simulink model "antywindup"  (R2019a)
settings: Solver=VariableStepAuto  StartTime=0.0  StopTime=50  RelTol=1e-3
values from neighbouring files (symbols this model uses):
  Kc = 10    [skrypt.m]
  Ki = 0.2    [skrypt.m]
  Kp = 2    [skrypt.m]
  u_sat = 10    [skrypt.m]
  y_ref = 10    [skrypt.m]
settings Model: Creator=szymo  LastModifiedBy=szymo

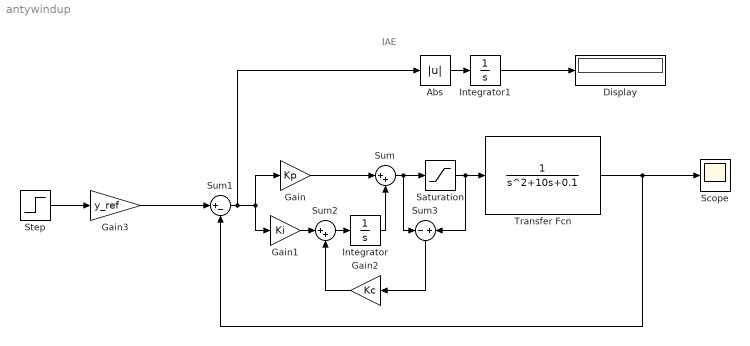
== system antywindup ==
  note: IAE
  Abs : Abs
  Display : Display
  Gain : Gain  Gain=Kp
  Gain1 : Gain  Gain=Ki
  Gain2 : Gain  Gain=Kc
  Gain3 : Gain  Gain=y_ref
  Integrator : Integrator
  Integrator1 : Integrator
  Saturation : Saturate  UpperLimit=u_sat  LowerLimit=-u_sat
  Scope : Scope
  Step : Step  SampleTime=0
  Sum : Sum  Inputs=|++
  Sum1 : Sum  Inputs=|+-
  Sum2 : Sum  Inputs=|++
  Sum3 : Sum  Inputs=-|+
  Transfer Fcn : TransferFcn  Denominator=[1 10 0.1]
  wires:
  Integrator/1 -> Sum/2
  Gain/1 -> Sum/1
  Sum/1 -> Sum3/1, Saturation/1
  Saturation/1 -> Sum3/2, Transfer Fcn/1
  Transfer Fcn/1 -> Sum1/2, Scope/1
  Gain3/1 -> Sum1/1
  Sum1/1 -> Abs/1, Gain1/1, Gain/1
  Abs/1 -> Integrator1/1
  Integrator1/1 -> Display/1
  Gain1/1 -> Sum2/1
  Sum2/1 -> Integrator/1
  Gain2/1 -> Sum2/2
  Sum3/1 -> Gain2/1
  Step/1 -> Gain3/1
